simulink model "ControlModel"  (R2018b)
settings: Solver=VariableStepAuto  StartTime=0.0  StopTime=10.0  RelTol=1e-3
libraries: cstblocks x5
settings Model: Creator=nikovertovec  LastModifiedBy=nikovertovec
settings DataIOCC: SaveFinalState=on  SaveState=on

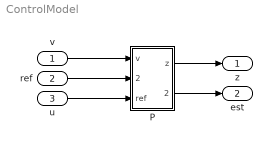
== system ControlModel ==
  v : Inport
  ref : Inport  Port=2
  u : Inport  Port=3
  P : Subsystem
  z : Outport
  est : Outport  Port=2
  wires:
  v/1 -> P/1(v)
  ref/1 -> P/2(noise)
  u/1 -> P/3(ref)
  P/1(z) -> z/1
  P/2(est) -> est/1

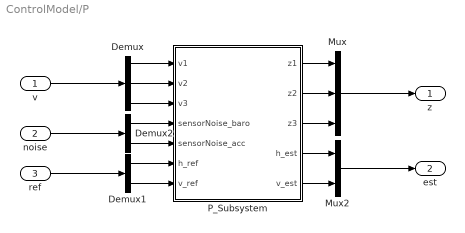
== system ControlModel/P ==
  v : Inport
  noise : Inport  Port=2
  ref : Inport  Port=3
  Demux : Demux  Outputs=3
  Demux1 : Demux  Outputs=2
  Demux2 : Demux  Outputs=2
  Mux : Mux  Inputs=3
  Mux2 : Mux  Inputs=2
  P_Subsystem : Subsystem
  z : Outport
  est : Outport  Port=2
  wires:
  Mux2/1 -> est/1
  Demux/1 -> P_Subsystem/1(v1)
  Demux1/1 -> P_Subsystem/6(h_ref)
  P_Subsystem/5(v_est) -> Mux2/2
  P_Subsystem/4(h_est) -> Mux2/1
  Demux1/2 -> P_Subsystem/7(v_ref)
  Demux/3 -> P_Subsystem/3(v3)
  P_Subsystem/3(z3) -> Mux/3
  P_Subsystem/2(z2) -> Mux/2
  Mux/1 -> z/1
  P_Subsystem/1(z1) -> Mux/1
  v/1 -> Demux/1
  Demux/2 -> P_Subsystem/2(v2)
  Demux2/2 -> P_Subsystem/5(sensorNoise_acc)
  Demux2/1 -> P_Subsystem/4(sensorNoise_baro)
  noise/1 -> Demux2/1
  ref/1 -> Demux1/1

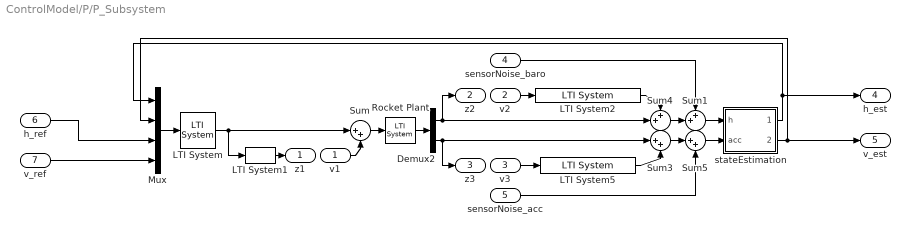
== system ControlModel/P/P_Subsystem ==
  v1 : Inport
  v2 : Inport  Port=2
  v3 : Inport  Port=3
  sensorNoise_baro : Inport  Port=4
  sensorNoise_acc : Inport  Port=5
  h_ref : Inport  Port=6
  v_ref : Inport  Port=7
  Demux2 : Demux  Outputs=2
  LTI System : cstblocks/LTI System  sys=Knom  IC=[]
  LTI System1 : cstblocks/LTI System  sys=Wu  IC=[]
  LTI System2 : cstblocks/LTI System  sys=W_inaccuracies_baro  IC=[]
  LTI System5 : cstblocks/LTI System  sys=W_inaccuracies_acc  IC=[]
  Mux : Mux
  Rocket Plant : cstblocks/LTI System  sys=G  IC=[]
  Sum : Sum  Inputs=|++  OutMin=0  OutMax=1
  Sum1 : Sum  Inputs=++|  OutMin=0  OutMax=1
  Sum3 : Sum  Inputs=|++  OutMin=0  OutMax=1
  Sum4 : Sum  Inputs=++|  OutMin=0  OutMax=1
  Sum5 : Sum  Inputs=|++  OutMin=0  OutMax=1
  stateEstimation : Subsystem
  z1 : Outport
  z2 : Outport  Port=2
  z3 : Outport  Port=3
  h_est : Outport  Port=4
  v_est : Outport  Port=5
  wires:
  v_ref/1 -> Mux/4
  Sum3/1 -> Sum5/1
  Sum1/1 -> stateEstimation/1(h)
  sensorNoise_baro/1 -> Sum1/1
  v2/1 -> LTI System2/1
  Sum4/1 -> Sum1/2
  v1/1 -> Sum/2
  stateEstimation/2(v_est) -> Mux/2, v_est/1
  LTI System/1 -> LTI System1/1, Sum/1
  sensorNoise_acc/1 -> Sum5/2
  LTI System1/1 -> z1/1
  Demux2/2 -> z3/1, Sum3/1
  Sum/1 -> Rocket Plant/1
  LTI System2/1 -> Sum4/1
  Rocket Plant/1 -> Demux2/1
  LTI System5/1 -> Sum3/2
  stateEstimation/1(h_est) -> h_est/1, Mux/1
  Demux2/1 -> z2/1, Sum4/2
  v3/1 -> LTI System5/1
  Sum5/1 -> stateEstimation/2(acc)
  Mux/1 -> LTI System/1
  h_ref/1 -> Mux/3

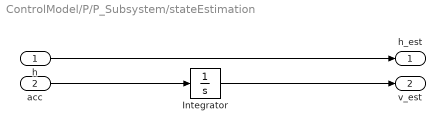
== system ControlModel/P/P_Subsystem/stateEstimation ==
  h : Inport
  acc : Inport  Port=2
  Integrator : Integrator
  h_est : Outport
  v_est : Outport  Port=2
  wires:
  acc/1 -> Integrator/1
  h/1 -> h_est/1
  Integrator/1 -> v_est/1
